simulink model "QArm_Workspace_MB_2"  (R2021a)
settings: Solver=ode4  StartTime=0.0  StopTime=inf  FixedStep=1/1000  RelTol=1e-3  EnableMultiTasking=on
model workspace (MAT data in the model file):
  cameraStepSize : Simulink.Parameter (value not decoded)
  mainStepSize : Simulink.Parameter (value not decoded)
symbols that are objects in the model workspace (value not decoded): cameraStepSize, mainStepSize
undefined symbols (not defined in the file): interleaved, RGB
libraries: quarc_library x12, simulink x3
(part 2 of 3)

== system QArm_Workspace_MB_2/Virtual QArm/Manipulator Joint Plants/Base Joint 1 ==
  note: v = IR + kv omega
      | Tau = i kt
      | Tau = J theta_dot_dot + b * omega + k *sign(omega)
  Voltage : Inport
  tau_g (Nm) : Inport  Port=2
  reset : Inport  Port=3
  Constant : Constant  Value=0.001*272.5
  Divide : Product  Inputs=*/
  Divide{1,3..5} (4 alike) : Product  Inputs=**
  Divide2 : Product  Inputs=*/
  Integrator1 : Integrator  ExternalReset=rising  LimitOutput=on  UpperSaturationLimit=pi*[170]/180  LowerSaturationLimit=pi*[-170]/180
  Integrator2 : Integrator  LimitOutput=on  UpperSaturationLimit=pi/2  LowerSaturationLimit=-pi/2
  J * GR^2 : Constant  Value=272.5^2*0.65e-05
  R : Constant
  Sign : Signum
  Subtract{,1..3} (4 alike) : Sum  Inputs=+-
  b * GR : Constant  Value=0.0005*272.5
  kt * GR : Constant  Value=0.01495*272.5
  kv * GR : Constant  Value=0.0135*272.5
  phi (rad) : Outport  VectorParamsAs1DForOutWhenUnconnected=off
  phi_dot (rad/s) : Outport  Port=2  VectorParamsAs1DForOutWhenUnconnected=off
  current (A) : Outport  Port=3  VectorParamsAs1DForOutWhenUnconnected=off
  wires:
  R/1 -> Divide/2
  Subtract/1 -> Divide/1
  kt * GR/1 -> Divide1/2
  Divide/1 -> current (A)/1, Divide1/1
  Divide3/1 -> Subtract/2
  Divide1/1 -> Subtract1/1
  J * GR^2/1 -> Divide2/2
  Voltage/1 -> Subtract/1
  kv * GR/1 -> Divide3/2
  b * GR/1 -> Divide4/2
  Integrator1/1 -> phi (rad)/1  "phi"
  Divide2/1 -> Integrator2/1
  Divide4/1 -> Subtract1/2
  Constant/1 -> Divide5/2
  Sign/1 -> Divide5/1
  Integrator2/1 -> Sign/1, Divide4/1, Divide3/1, Integrator1/1, phi_dot (rad/s)/1  "Speed"
  Subtract1/1 -> Subtract2/1
  Divide5/1 -> Subtract2/2
  Subtract2/1 -> Subtract3/1
  Subtract3/1 -> Divide2/1
  tau_g (Nm)/1 -> Subtract3/2
  reset/1 -> Integrator1/2

== system QArm_Workspace_MB_2/Virtual QArm/Manipulator Joint Plants/Elbow Joint 3 ==
  Voltage : Inport
  tau_g (Nm) : Inport  Port=2
  reset : Inport  Port=3
  Constant : Constant  Value=0.001*272.5
  Divide : Product  Inputs=*/
  Divide{1,3..5} (4 alike) : Product  Inputs=**
  Divide2 : Product  Inputs=*/
  Integrator1 : Integrator  ExternalReset=rising  LimitOutput=on  UpperSaturationLimit=pi*[75]/180  LowerSaturationLimit=pi*[-95]/180
  Integrator2 : Integrator  LimitOutput=on  UpperSaturationLimit=pi/2  LowerSaturationLimit=-pi/2
  J * GR^2 : Constant  Value=272.5^2*0.75e-05
  R : Constant  Value=5
  Sign : Signum
  Subtract{,1..3} (4 alike) : Sum  Inputs=+-
  b * GR : Constant  Value=0.02*272.5
  kt * GR : Constant  Value=0.1*272.5
  kv * GR : Constant  Value=0.01*272.5
  phi (rad) : Outport  VectorParamsAs1DForOutWhenUnconnected=off
  phi_dot (rad/s) : Outport  Port=2  VectorParamsAs1DForOutWhenUnconnected=off
  current (A) : Outport  Port=3  VectorParamsAs1DForOutWhenUnconnected=off
  wires:
  R/1 -> Divide/2
  Subtract/1 -> Divide/1
  kt * GR/1 -> Divide1/2
  Divide/1 -> current (A)/1, Divide1/1
  Integrator2/1 -> Divide4/1, Divide3/1, Sign/1, phi_dot (rad/s)/1, Integrator1/1  "Speed"
  Divide3/1 -> Subtract/2
  Divide1/1 -> Subtract1/1
  J * GR^2/1 -> Divide2/2
  Subtract1/1 -> Subtract2/1
  Voltage/1 -> Subtract/1
  kv * GR/1 -> Divide3/2
  b * GR/1 -> Divide4/2
  Integrator1/1 -> phi (rad)/1  "phi"
  Divide2/1 -> Integrator2/1
  Divide4/1 -> Subtract1/2
  Divide5/1 -> Subtract2/2
  Constant/1 -> Divide5/2
  Sign/1 -> Divide5/1
  Subtract3/1 -> Divide2/1
  Subtract2/1 -> Subtract3/1
  tau_g (Nm)/1 -> Subtract3/2
  reset/1 -> Integrator1/2

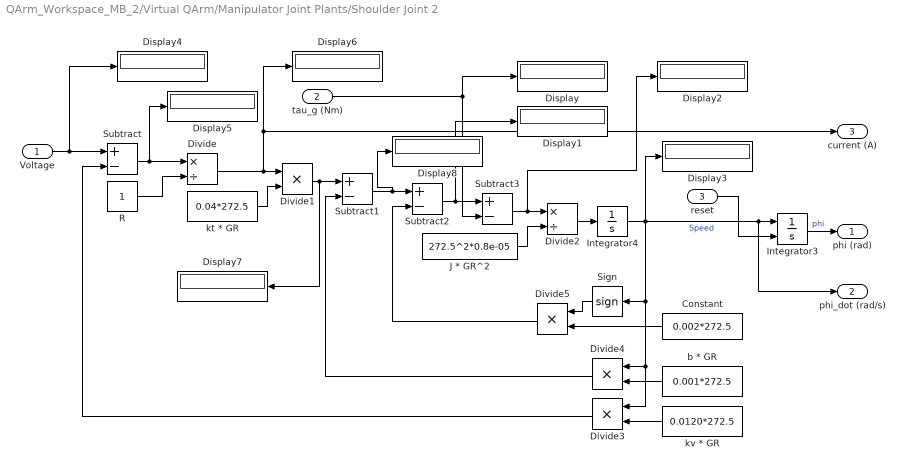
== system QArm_Workspace_MB_2/Virtual QArm/Manipulator Joint Plants/Shoulder Joint 2 ==
  Voltage : Inport
  tau_g (Nm) : Inport  Port=2
  reset : Inport  Port=3
  Constant : Constant  Value=0.002*272.5
  Display{,1..8} (9 alike) : Display
  Divide : Product  Inputs=*/
  Divide{1,3..5} (4 alike) : Product  Inputs=**
  Divide2 : Product  Inputs=*/
  Integrator3 : Integrator  ExternalReset=rising  LimitOutput=on  UpperSaturationLimit=pi*[85]/180  LowerSaturationLimit=pi*[-85]/180
  Integrator4 : Integrator  LimitOutput=on  UpperSaturationLimit=pi/2  LowerSaturationLimit=-pi/2
  J * GR^2 : Constant  Value=272.5^2*0.8e-05
  R : Constant
  Sign : Signum
  Subtract{,1..3} (4 alike) : Sum  Inputs=+-
  b * GR : Constant  Value=0.001*272.5
  kt * GR : Constant  Value=0.04*272.5
  kv * GR : Constant  Value=0.0120*272.5
  phi (rad) : Outport  VectorParamsAs1DForOutWhenUnconnected=off
  phi_dot (rad/s) : Outport  Port=2  VectorParamsAs1DForOutWhenUnconnected=off
  current (A) : Outport  Port=3  VectorParamsAs1DForOutWhenUnconnected=off
  wires:
  Divide4/1 -> Subtract1/2
  Divide2/1 -> Integrator4/1
  Integrator3/1 -> phi (rad)/1  "phi"
  b * GR/1 -> Divide4/2
  kv * GR/1 -> Divide3/2
  Voltage/1 -> Display4/1, Subtract/1
  Subtract1/1 -> Display8/1, Subtract2/1
  J * GR^2/1 -> Divide2/2
  Divide1/1 -> Subtract1/1, Display7/1
  Divide3/1 -> Subtract/2
  Divide/1 -> Divide1/1, Display6/1, current (A)/1
  kt * GR/1 -> Divide1/2
  Subtract/1 -> Display5/1, Divide/1
  R/1 -> Divide/2
  Constant/1 -> Divide5/2
  Sign/1 -> Divide5/1
  Integrator4/1 -> Display3/1, Integrator3/1, phi_dot (rad/s)/1, Sign/1, Divide3/1, Divide4/1  "Speed"
  Divide5/1 -> Subtract2/2
  Subtract3/1 -> Display2/1, Divide2/1
  Subtract2/1 -> Display1/1, Subtract3/1
  tau_g (Nm)/1 -> Subtract3/2, Display/1
  reset/1 -> Integrator3/2

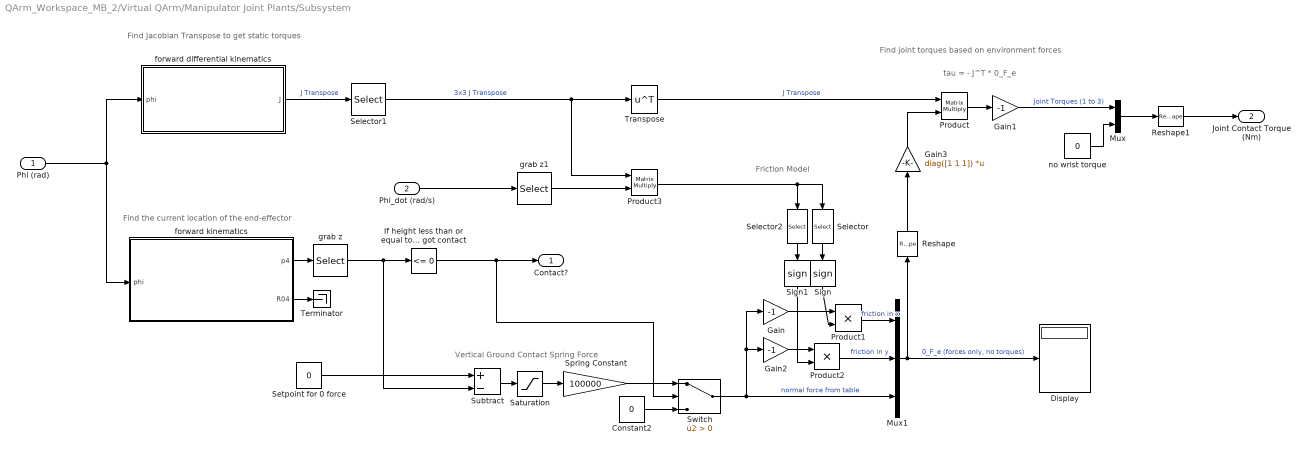
== system QArm_Workspace_MB_2/Virtual QArm/Manipulator Joint Plants/Subsystem ==
  note: Friction Model
  note: Vertical Ground Contact Spring Force
  note: Find joint torques based on environment forces
  note: Find Jacobian Transpose to get static torques
  note: Find the current location of the end-effector
  note: tau = - J^T * 0_F_e
  Phi (rad) : Inport  PortDimensions=4
  Phi_dot (rad/s) : Inport  Port=2  PortDimensions=4
  Constant2 : Constant  Value=0
  Display : Display
  Gain : Gain  Gain=-1
  Gain1 : Gain  Gain=-1
  Gain2 : Gain  Gain=-1
  Gain3 : Gain  Gain=diag([1 1 1])  Multiplication=Matrix(K*u)
  "If height less than or equal to 0, then we've got contact" : simulink/Logic and Bit Operations/Compare To Constant  relop=<=  const=0  OutDataTypeStr=boolean
  Mux : Mux  Inputs=2
  Mux1 : Mux  Inputs=3
  Product : Product  Multiplication=Matrix(*)
  Product1 : Product
  Product2 : Product
  Product3 : Product  Multiplication=Matrix(*)
  Reshape : Reshape  OutputDimensionality=Column vector (2-D)
  Reshape1 : Reshape
  Saturation : Saturate  UpperLimit=Inf  LowerLimit=0
  Selector : Selector  InputPortWidth=3  IndexOptions=Index vector (dialog)  Indices=1  OutputSizes=1
  Selector1 : Selector  NumberOfDimensions=2  InputPortWidth=3  IndexOptions=Index vector (dialog),Index vector (dialog)  Indices=[1:3],[1:3]  OutputSizes=1,1
  Selector2 : Selector  InputPortWidth=3  IndexOptions=Index vector (dialog)  Indices=2  OutputSizes=1
  Setpoint for 0 force : Constant  Value=0
  Sign : Signum
  Sign1 : Signum
  Spring Constant : Gain  Gain=100000
  Subtract : Sum  Inputs=+-
  Switch : Switch  Criteria=u2 > Threshold
  Terminator : Terminator
  Transpose : Math  Operator=transpose  SignedPower=on  SaturateOnIntegerOverflow=on
  forward differential kinematics : MATLAB Function  TreatAsAtomicUnit=on
  forward kinematics : MATLAB Function  TreatAsAtomicUnit=on
  grab z : Selector  InputPortWidth=3  IndexOptions=Index vector (dialog)  Indices=3  OutputSizes=1
  grab z1 : Selector  InputPortWidth=4  IndexOptions=Index vector (dialog)  Indices=[1:3]  OutputSizes=1
  no wrist torque : Constant  Value=0
  Contact? : Outport  VectorParamsAs1DForOutWhenUnconnected=off
  Joint Contact Torque (Nm) : Outport  Port=2  VectorParamsAs1DForOutWhenUnconnected=off
  wires:
  forward kinematics/1(p4) -> grab z/1
  forward kinematics/2(R04) -> Terminator/1
  grab z/1 -> "If height less than or equal to 0, then we've got contact"/1, Subtract/2
  forward differential kinematics/1(J) -> Selector1/1  "J Transpose"
  Mux1/1 -> Reshape/1, Display/1  "0_F_e (forces only, no torques)"
  Selector1/1 -> Product3/1, Transpose/1  "3x3 J Transpose"
  Product/1 -> Gain1/1
  no wrist torque/1 -> Mux/2
  Mux/1 -> Reshape1/1
  Gain1/1 -> Mux/1  "Joint Torques (1 to 3)"
  Switch/1 -> Mux1/3, Gain2/1, Gain/1  "normal force from table"
  Product2/1 -> Mux1/2  "friction in y"
  "If height less than or equal to 0, then we've got contact"/1 -> Contact?/1, Switch/2
  Constant2/1 -> Switch/3
  Spring Constant/1 -> Switch/1
  Setpoint for 0 force/1 -> Subtract/1
  Subtract/1 -> Saturation/1
  Phi (rad)/1 -> forward differential kinematics/1(phi), forward kinematics/1(phi)
  Reshape/1 -> Gain3/1
  Reshape1/1 -> Joint Contact Torque (Nm)/1
  Product1/1 -> Mux1/1  "friction in x"
  Saturation/1 -> Spring Constant/1
  Phi_dot (rad/s)/1 -> grab z1/1
  Product3/1 -> Selector2/1, Selector/1
  Gain/1 -> Product1/1
  Gain2/1 -> Product2/1
  Selector/1 -> Sign/1
  Selector2/1 -> Sign1/1
  Gain3/1 -> Product/2
  Sign/1 -> Product1/2
  Sign1/1 -> Product2/2
  Transpose/1 -> Product/1  "J Transpose"
  grab z1/1 -> Product3/2

== system QArm_Workspace_MB_2/Virtual QArm/Manipulator Joint Plants/Wrist Joint 4 ==
  Voltage : Inport
  tau_g (Nm) : Inport  Port=2
  reset : Inport  Port=3
  Constant : Constant  Value=0.001*272.5
  Divide : Product  Inputs=*/
  Divide{1,3..5} (4 alike) : Product  Inputs=**
  Divide2 : Product  Inputs=*/
  Integrator3 : Integrator  ExternalReset=rising  LimitOutput=on  UpperSaturationLimit=pi*[167.5]/180  LowerSaturationLimit=pi*[-167.5]/180
  Integrator4 : Integrator  LimitOutput=on  UpperSaturationLimit=pi  LowerSaturationLimit=-pi
  J * GR^2 : Constant  Value=272.5^2*0.5e-05
  R : Constant  Value=6
  Sign : Signum
  Subtract{,1..3} (4 alike) : Sum  Inputs=+-
  b * GR : Constant  Value=0.001*272.5
  kt * GR : Constant  Value=0.3*272.5
  kv * GR : Constant  Value=0.0095*272.5
  phi (rad) : Outport  VectorParamsAs1DForOutWhenUnconnected=off
  phi_dot (rad/s) : Outport  Port=2  VectorParamsAs1DForOutWhenUnconnected=off
  current (A) : Outport  Port=3  VectorParamsAs1DForOutWhenUnconnected=off
  wires:
  Divide4/1 -> Subtract1/2
  Divide2/1 -> Integrator4/1
  Integrator3/1 -> phi (rad)/1  "phi"
  b * GR/1 -> Divide4/2
  kv * GR/1 -> Divide3/2
  Voltage/1 -> Subtract/1
  Subtract1/1 -> Subtract2/1
  J * GR^2/1 -> Divide2/2
  Divide1/1 -> Subtract1/1
  Divide3/1 -> Subtract/2
  Divide/1 -> Divide1/1, current (A)/1
  kt * GR/1 -> Divide1/2
  Subtract/1 -> Divide/1
  R/1 -> Divide/2
  Sign/1 -> Divide5/1
  Constant/1 -> Divide5/2
  Integrator4/1 -> Integrator3/1, phi_dot (rad/s)/1, Sign/1, Divide3/1, Divide4/1  "Speed"
  Divide5/1 -> Subtract2/2
  Subtract3/1 -> Divide2/1
  Subtract2/1 -> Subtract3/1
  tau_g (Nm)/1 -> Subtract3/2
  reset/1 -> Integrator3/2

== matlab function QArm_Workspace_MB_2/To//From Simulation/MATLAB Function4 ==
  settings: updateMethod=DISCRETE  sampleTime=mainStepSize
  data: Packet output size=65537; ServerState input; SendStateUpdate input; Enable output; DeviceNumber input; Clock input; Threshold input
function [Packet,Enable] = QArmApplicationWorkspaceMakeVideoPacketData(ServerState, SendStateUpdate, DeviceNumber, Clock, Threshold) 

% Be sure to set the maximum signal size of the variable size Packet port 
% in Simulink->Edit Data of the editor window.  Size should be 65537 or
% larger to ensure that the stream server generates a 4 byte packet size.

%% Setup
persistent LastServerState;
persistent timeLastSend;
persistent readyToSend;

if isempty(LastServerState)
    LastServerState = uint8(0);
    readyToSend = uint8(0);
    timeLastSend = -Threshold;
end

Enable = 0;
Packet = uint8([]);

%% On connection
if ((ServerState == 2) && (LastServerState ~= 2))
    Packet = QArmMakeRGBRawRequestContainer(DeviceNumber);
    Packet = [Packet; QArmMakeDepthRawRequestContainer(DeviceNumber)];
end

%% Send new State Container
% Previous state processed, send a new one
if (SendStateUpdate)
    readyToSend = uint8(1);
end

if readyToSend && ((Clock - timeLastSend) > Threshold)
    Packet = QArmMakeRGBRawRequestContainer(DeviceNumber);
    Packet = [Packet; QArmMakeDepthRawRequestContainer(DeviceNumber)];   
    readyToSend = uint8(0);
    timeLastSend = Clock;
end


%% Transmit
% If we have data to send, enable the transmit
PacketLength = length(Packet);

if (PacketLength > 0)
    % Add magic byte.  This is just for error handling and isn't typically
    % required in simulink, but useful in lower-level languages like Python
    Packet = [uint8(123); Packet];
    
    Enable = 1; 
end

LastServerState = ServerState;

== matlab function QArm_Workspace_MB_2/Virtual QArm/Manipulator Joint Plants/Gravitational Torque ==
  data: phi input; G output; payload input
function G  = fcn(phi, payload)

%% Manipulator Parameters and Initialization

% Manipulator natural link lengths
L1 = 0.1400;
L2 = 0.3500;
L3 = 0.0500;
L4 = 0.2500;
L5 = 0.1500;

% Manipulator bend angle at joint 3
beta = atan(L3/L2);

% Manipulator mathematical link lenghts
l1 = L1;
l2 = sqrt(L2^2 + L3^2);
l3 = L4 + L5;

% Phi-space to Theta-space
theta = phi;
theta(1) = phi(1);
theta(2) = phi(2) + beta - pi/2;
theta(3) = phi(3) - beta;
theta(4) = phi(4);

%% Dynamic Parameters (Inertias and Masses)

% Masses
mT = 1.75;
m1 = 0.3*mT*l1 / (l1 + l2 + l3);
m2 = mT*l2 / (l1 + l2 + l3);
m3 = mT*L4 / (l1 + l2 + l3);
m4 = mT*L5 / (l1 + l2 + l3);
mL = payload;

% Center of mass locations
% Note: lc1 is unused as the first link does not move linearly (v_1 = 0)
lc2 = l2/2;
lc3 = L4/2;
lc4 = L5/2;

%% Gravity Matrix

g = 9.81;
G2 = -g*(m2*(l2 - lc2)*cos(theta(2)) + m3*(l2*cos(theta(2)) - lc3*sin(theta(2)+theta(3))) + m4*(l2*cos(theta(2)) - (l3 - lc4)*sin(theta(2)+theta(3))) + mL*(l2*cos(theta(2)) - l3*sin(theta(2)+theta(3))) );
G3 = g*(m3*lc3*sin(theta(2)+theta(3)) + m4*(l3 - lc4)*sin(theta(2)+theta(3)) + mL*l3*sin(theta(2)+theta(3)) );

G = [0; G2; G3; 0];

== matlab function QArm_Workspace_MB_2/To//From Simulation/MATLAB Function5 ==
  data: Receive input; RequestServerUpdate output; NewRGB output; New input; RGB output; NewDepth output; Depth output
function [RequestServerUpdate, NewRGB, RGB, NewDepth, Depth]  = QArmApplicationWorkspaceDecodeVideoPacket(Receive, New)

%% Setup

num_columns = 1280;
num_rows = 720;

RGB = zeros(num_rows*num_columns*3, 1, 'uint8');
Depth = zeros(num_rows*num_columns*3, 1, 'uint8');

NewRGB = 0;
NewDepth = 0;

RequestServerUpdate = 0;
PacketSize = length(Receive);

%Packet > 0, new data, and magic number in first index
if ((PacketSize > 0) && (New == 1) && (Receive(1) == uint8(123)))
    
    %skip magic number
    Index = int32(2);
    
    while(Index <= PacketSize)
       
        %% Get container details
        ContainerSize = typecast(uint8(flip(Receive(Index:Index+3))), 'int32');
        DeviceID = typecast(uint8(flip(Receive(Index+4:Index+7))), 'int32');
        DeviceNum = typecast(uint8(flip(Receive(Index+8:Index+12))), 'int32');
        DeviceFunction = uint8(Receive(Index+12));
        PayloadStart = Index+13;
        PayloadEnd = Index+ContainerSize-1;
        
        %% Pass container to appropriate decoding function
        if (DeviceID == 10) %is this a QArm container?
            
            if (DeviceFunction == 103) % Pull out RGB payload for external processing
                RGBSize = typecast(uint8(flip(Receive(PayloadStart:PayloadStart+3))), 'int32');
                RGB(1:num_rows*num_columns*3) = Receive(PayloadStart+4:PayloadStart+4+num_rows*num_columns*3);
                NewRGB = 1;
                RequestServerUpdate = 1;
                
            elseif (DeviceFunction == 113) % Pull out Depth payload for external processing
                DepthSize = typecast(uint8(flip(Receive(PayloadStart:PayloadStart+3))), 'int32');
                Depth(1:num_rows*num_columns*3) = Receive(PayloadStart+4:PayloadStart+4+num_rows*num_columns*3);
                NewDepth = 1;
                RequestServerUpdate = 1;
            end
        end
        
        
        
        %% Process next container if any data is left.
        Index = Index+ContainerSize;
    end


end

== matlab function QArm_Workspace_MB_2/To//From Simulation/MATLAB Function3 ==
  data: Receive input size=65537; RequestServerUpdate output; NewRGB output; New input; RGB output size=65537; NewDepth output; Depth output size=65537
function [RequestServerUpdate, NewRGB, RGB, NewDepth, Depth]  = QArmApplicationWorkspaceDecodeVideoPacket(Receive, New)

%% Setup
RGB = uint8([]);
Depth = uint8([]);

NewRGB = 0;
NewDepth = 0;

RequestServerUpdate = 0;
PacketSize = length(Receive);

% Packet > 0, new data, and magic number in first index
if ((PacketSize > 0) && (New == 1) && (Receive(1) == uint8(123)))
    
    %skip magic number
    Index = int32(2);
    
    while(Index <= PacketSize)
       
                %% Get container details
        ContainerSize = typecast(uint8(flip(Receive(Index:Index+3))), 'int32');
        DeviceID = typecast(uint8(flip(Receive(Index+4:Index+7))), 'int32');
        DeviceNum = typecast(uint8(flip(Receive(Index+8:Index+11))), 'int32');
        DeviceFunction = uint8(Receive(Index+12));
        PayloadStart = Index+13;
        PayloadEnd = Index+ContainerSize-1;
        
        %% Pass container to appropriate decoding function
        if (DeviceID == 10) %is this a QArm container?
            
            if (DeviceFunction == 2) % Pull out RGB payload for external processing
                RequestServerUpdate = 1;
            
            elseif (DeviceFunction == 101) % Pull out RGB payload for external processing
                RGBSize = typecast(uint8(flip(Receive(PayloadStart:PayloadStart+3))), 'int32');
                RGB = Receive(PayloadStart+4:PayloadEnd);
                NewRGB = 1;
                RequestServerUpdate = 1;
                
            elseif (DeviceFunction == 111) % Pull out Depth payload for external processing
                DepthSize = typecast(uint8(flip(Receive(PayloadStart:PayloadStart+3))), 'int32');
                Depth = Receive(PayloadStart+4:PayloadEnd);
                NewDepth = 1;
                RequestServerUpdate = 1;
            end
        end
        
        
        
        %% Process next container if any data is left.
        Index = Index+ContainerSize;
    end


end

== matlab function QArm_Workspace_MB_2/To//From Simulation/Collision/inverse kinematics ==
  data: p input; gamma input; phi_optimal output; phi_prev input
function phi_optimal  = qarmInverseKinematics(p, gamma, phi_prev)

%% QUANSER_ARM_IPK
% v 4.0 - 4th June 2020

% REFERENCE: 
% Chapter 4. Inverse Kinematics
% Robot Dynamics and Control 
% Spong, Vidyasagar
% 1989

% INPUTS:
% p        : end-effector position vector expressed in base frame {0}
% gamma    : wrist rotation angle gamma

% OUTPUTS:
% phi_optimal : Best solution depending on phi_prev
% phi         : All four Inverse Kinematics solutions as a 4x4 matrix. 
%               Each col is a solution.

%% Manipulator parameters:
L1 = 0.1400;
L2 = 0.3500;
L3 = 0.0500;
L4 = 0.2500;
L5 = 0.1500;
beta = atan(L3/L2);

%% Alternate parameters
lambda1 = L1;
lambda2 = sqrt(L2^2 + L3^2);
lambda3 = L4 + L5;

%% Initialization
theta   = zeros(4, 4);
phi = zeros(4, 4);

%% Joint angle 2 and 3: 
% Equations:
    % lambda2 cos(theta2) + (-lambda3) sin(theta2 + theta3) = sqrt(x^2 + y^2)
    %   A     cos( 2    ) +     C      sin(   2   +    3  ) =    D
    
    % lambda2 sin(theta2) - (-lambda3) cos(theta2 + theta3) = lambda1 - z
    %   A     sin( 2    ) -     C      cos(   2   +    3  ) =    H

% Solution:
    A = lambda2;
    C = -lambda3;
    H =  lambda1 - p(3);
    D1 = -sqrt(p(1)^2 + p(2)^2);
    D2 = sqrt(p(1)^2 + p(2)^2);
    F = (D1^2 + H^2 - A^2 - C^2)/(2*A);

    theta(3,1) = 2*atan2( C + sqrt(C^2 - F^2) , F );
	theta(3,2) = 2*atan2( C - sqrt(C^2 - F^2) , F );
    theta(3,3) = 2*atan2( C + sqrt(C^2 - F^2) , F );
	theta(3,4) = 2*atan2( C - sqrt(C^2 - F^2) , F );

    M = A + C*sin(theta(3,1));
    N = -C*cos(theta(3,1));
    cos_term = (D1*M + H*N)/(M^2 + N^2);
    sin_term = (H - N*cos_term)/(M);
    theta(2,1) = atan2(sin_term, cos_term);

    M = A + C*sin(theta(3,2));
    N = -C*cos(theta(3,2));
    cos_term = (D1*M + H*N)/(M^2 + N^2);
    sin_term = (H - N*cos_term)/(M);
    theta(2,2) = atan2(sin_term, cos_term);

    M = A + C*sin(theta(3,3));
    N = -C*cos(theta(3,3));
    cos_term = (D2*M + H*N)/(M^2 + N^2);
    sin_term = (H - N*cos_term)/(M);
    theta(2,3) = atan2(sin_term, cos_term);

    M = A + C*sin(theta(3,4));
    N = -C*cos(theta(3,4));
    cos_term = (D2*M + H*N)/(M^2 + N^2);
    sin_term = (H - N*cos_term)/(M);
    theta(2,4) = atan2(sin_term, cos_term);


%% Joint angle 1:
% Equation:
    % y / x = tan(theta1);

% Solution
    theta(1,1) = atan2( p(2)/( lambda2 * cos( theta(2,1) ) - lambda3 * sin( theta(2,1) + theta(3,1) ) ) , p(1)/(  lambda2 * cos( theta(2,1) ) - lambda3 * sin( theta(2,1) + theta(3,1) )  ) );
    theta(1,2) = atan2( p(2)/( lambda2 * cos( theta(2,2) ) - lambda3 * sin( theta(2,2) + theta(3,2) ) ) , p(1)/(  lambda2 * cos( theta(2,2) ) - lambda3 * sin( theta(2,2) + theta(3,2) )  ) );
    theta(1,3) = atan2( p(2)/( lambda2 * cos( theta(2,3) ) - lambda3 * sin( theta(2,3) + theta(3,3) ) ) , p(1)/(  lambda2 * cos( theta(2,3) ) - lambda3 * sin( theta(2,3) + theta(3,3) )  ) );
    theta(1,4) = atan2( p(2)/( lambda2 * cos( theta(2,4) ) - lambda3 * sin( theta(2,4) + theta(3,4) ) ) , p(1)/(  lambda2 * cos( theta(2,4) ) - lambda3 * sin( theta(2,4) + theta(3,4) )  ) );
    
%% Remap theta back to phi
% phi(1) = theta(1);
% phi(2) = theta(2) - beta + pi/2;
% phi(3) = theta(3) + beta;
% phi(4) = theta(4);

phi(1,:) = theta(1,:);
phi(2,:) = theta(2,:) - beta + pi/2;
phi(3,:) = theta(3,:) + beta;
phi(4,:) = gamma;

phi = mod(phi + pi, 2*pi) - pi;

phi_optimal = phi(:,1);
if norm(phi_optimal - phi_prev) > norm(phi(:,2) - phi_prev)
    phi_optimal = phi(:,2);
end
if norm(phi_optimal - phi_prev) > norm(phi(:,3) - phi_prev)
    phi_optimal = phi(:,3);
end
if norm(phi_optimal - phi_prev) > norm(phi(:,4) - phi_prev)
    phi_optimal = phi(:,4);
end

end

== matlab function QArm_Workspace_MB_2/To//From Simulation/Collision/MATLAB Function ==
  settings: updateMethod=DISCRETE
  data: user_phi input; user_p input; position_cmd output; target input; actual input; R04 input; where output; offset input
function [position_cmd, where] = fcn(user_phi, user_p, target, actual, R04, offset)

persistent state
persistent phi
persistent p
persistent actual_hold
change = 0; collision = 0;

if isempty(state)
    state = 1;
    phi = user_phi;
    actual_hold = actual;
end

if norm(user_phi-phi, 2) > 0.001
    change = 1;
end

if norm(target-actual, 2) > 0.001
    collision = 1;
end

switch state
    case 1
        if collision
            state = 2;
        else
            state = 1;
        end
        p = user_p;
        
    case 2
        state = 3;
        actual_hold = actual;
        p = actual_hold - R04*offset;
        
    case 3
        if change
            state = 1;
        else
            state = 3;
        end      
        
        p = actual_hold - R04*offset;
        
    otherwise
        p = user_p;
end

phi = user_phi;
position_cmd = p;
where = state;

== matlab function QArm_Workspace_MB_2/To//From Simulation/Collision/forward kinematics1 ==
  data: phi input; p4 output; R04 output
function [p4, R04] = qarmForwardKinematics(phi)

%% QUANSER_ARM_FPK
% v 4.0 - 4th June 2020

% REFERENCE: 
% Chapter 3. Forward Kinematics
% Robot Dynamics and Control 
% Spong, Vidyasagar
% 1989

% INPUTS:
% phi     : Alternate joint angles vector 4 x 1

% OUTPUTS:
% p4      : End-effector frame {4} position vector expressed in base frame {0}
% R04     : rotation matrix from end-effector frame {4} to base frame {0}

%% Manipulator parameters:
L1 = 0.1400;
L2 = 0.3500;
L3 = 0.0500;
L4 = 0.2500;
L5 = 0.1500;

%% Alternate parameters
l1 = L1;
l2 = sqrt(L2^2 + L3^2);
l3 = L4 + L5;
beta = atan(L3/L2);

%% From phi space to theta space 
theta = phi;
theta(1) = phi(1);
theta(2) = phi(2) + beta - pi/2;
theta(3) = phi(3) - beta;
theta(4) = phi(4);

%% Transformation matrices for all frames:

% T{i-1}{i} = quanser_arm_DH(  a, alpha,  d,     theta );
        T01 = quanser_arm_DH(  0, -pi/2, l1,  theta(1) );
        T12 = quanser_arm_DH( l2,     0,  0,  theta(2) );
        T23 = quanser_arm_DH(  0, -pi/2,  0,  theta(3) );
        T34 = quanser_arm_DH(  0,     0, l3,  theta(4) );

        T02 = T01*T12;
        T03 = T02*T23;
        T04 = T03*T34;

%% Position of end-effector Transformation

% Extract the Position vector 
% p1   = T01(1:3,4);
% p2   = T02(1:3,4);
% p3   = T03(1:3,4);
p4   = T04(1:3,4);

% Extract the Rotation matrix
% R01 = T01(1:3,1:3);
% R02 = T02(1:3,1:3);
% R03 = T03(1:3,1:3);
R04 = T04(1:3,1:3);

end

function T = quanser_arm_DH(a,alpha,d,theta)

%% QUANSER_ARM_DH
% v 1.0 - 26th March 2019

% REFERENCE: 
% Chapter 3. Forward and Inverse Kinematics
% Robot Modeling and Control 
% Spong, Hutchinson, Vidyasagar
% 2006

% INPUTS:
% a       :   translation  : along : x_{i}   : from : z_{i-1} : to : z_{i}
% alpha   :      rotation  : about : x_{i}   : from : z_{i-1} : to : z_{i}
% d       :   translation  : along : z_{i-1} : from : x_{i-1} : to : x_{i}
% theta   :      rotation  : about : z_{i-1} : from : x_{i-1} : to : x_{i}
% NOTE: Standard DH Parameters

% OUTPUTS:
% T       : transformation                   : from :     {i} : to : {i-1}

%%
% Rotation Transformation about z axis by theta
T_R_z = [cos(theta) -sin(theta) 0 0;
         sin(theta)  cos(theta) 0 0;
                  0           0 1 0;
                  0           0 0 1];
     
% Translation Transformation along z axis by d
T_T_z = [1 0 0 0;
         0 1 0 0;
         0 0 1 d;
         0 0 0 1];

% Translation Transformation along x axis by a
T_T_x = [1 0 0 a;
         0 1 0 0;
         0 0 1 0;
         0 0 0 1];

% Rotation Transformation about x axis by alpha
T_R_x = [1          0           0 0;
         0 cos(alpha) -sin(alpha) 0;
         0 sin(alpha)  cos(alpha) 0;
         0          0           0 1];

% For a transformation FROM frame {i} TO frame {i-1}: A
T = T_R_z*T_T_z*T_T_x*T_R_x;

end

== matlab function QArm_Workspace_MB_2/To//From Simulation/Collision (Archive)/MATLAB Function ==
  data: user_phi input; user_p input; position_cmd output; target input; actual input; R04 input
function position_cmd = fcn(user_phi, user_p, target, actual, R04)

persistent state
persistent phi
persistent p
persistent actual_hold
change = 0; collision = 0;

if isempty(state)
    state = 1;
    phi = user_phi;
    p = user_p;
    actual_hold = actual;
end

if user_phi ~= phi
    change = 1;
end

if target ~= actual
    collision = 1;
end

switch state
    case 1
        if collision
            state = 2;
        else
            state = 1;
        end
        p = user_p;
        
    case 2
        state = 3;
        actual_hold = actual;
        p = actual_hold - R04*[-0.0256;0;-0.1162];
        
    case 3
        if change
            state = 1;
        else
            state = 3;
        end      
        
        p = actual_hold - R04*[-0.0256;0;-0.1162];
        
    otherwise
        p = user_p;
end

phi = user_phi;
position_cmd = p;

== matlab function QArm_Workspace_MB_2/To//From Simulation/Collision (Archive)/forward kinematics ==
  data: phi input; p4 output; R04 output
function [p4, R04] = qarmForwardKinematics(phi)

%% QUANSER_ARM_FPK
% v 4.0 - 4th June 2020

% REFERENCE: 
% Chapter 3. Forward Kinematics
% Robot Dynamics and Control 
% Spong, Vidyasagar
% 1989

% INPUTS:
% phi     : Alternate joint angles vector 4 x 1

% OUTPUTS:
% p4      : End-effector frame {4} position vector expressed in base frame {0}
% R04     : rotation matrix from end-effector frame {4} to base frame {0}

%% Manipulator parameters:
L1 = 0.1400;
L2 = 0.3500;
L3 = 0.0500;
L4 = 0.2500;
L5 = 0.1500;

%% Alternate parameters
l1 = L1;
l2 = sqrt(L2^2 + L3^2);
l3 = L4 + L5;
beta = atan(L3/L2);

%% From phi space to theta space 
theta = phi;
theta(1) = phi(1);
theta(2) = phi(2) + beta - pi/2;
theta(3) = phi(3) - beta;
theta(4) = phi(4);

%% Transformation matrices for all frames:

% T{i-1}{i} = quanser_arm_DH(  a, alpha,  d,     theta );
        T01 = quanser_arm_DH(  0, -pi/2, l1,  theta(1) );
        T12 = quanser_arm_DH( l2,     0,  0,  theta(2) );
        T23 = quanser_arm_DH(  0, -pi/2,  0,  theta(3) );
        T34 = quanser_arm_DH(  0,     0, l3,  theta(4) );

        T02 = T01*T12;
        T03 = T02*T23;
        T04 = T03*T34;

%% Position of end-effector Transformation

% Extract the Position vector 
% p1   = T01(1:3,4);
% p2   = T02(1:3,4);
% p3   = T03(1:3,4);
p4   = T04(1:3,4);

% Extract the Rotation matrix
% R01 = T01(1:3,1:3);
% R02 = T02(1:3,1:3);
% R03 = T03(1:3,1:3);
R04 = T04(1:3,1:3);

end

function T = quanser_arm_DH(a,alpha,d,theta)

%% QUANSER_ARM_DH
% v 1.0 - 26th March 2019

% REFERENCE: 
% Chapter 3. Forward and Inverse Kinematics
% Robot Modeling and Control 
% Spong, Hutchinson, Vidyasagar
% 2006

% INPUTS:
% a       :   translation  : along : x_{i}   : from : z_{i-1} : to : z_{i}
% alpha   :      rotation  : about : x_{i}   : from : z_{i-1} : to : z_{i}
% d       :   translation  : along : z_{i-1} : from : x_{i-1} : to : x_{i}
% theta   :      rotation  : about : z_{i-1} : from : x_{i-1} : to : x_{i}
% NOTE: Standard DH Parameters

% OUTPUTS:
% T       : transformation                   : from :     {i} : to : {i-1}

%%
% Rotation Transformation about z axis by theta
T_R_z = [cos(theta) -sin(theta) 0 0;
         sin(theta)  cos(theta) 0 0;
                  0           0 1 0;
                  0           0 0 1];
     
% Translation Transformation along z axis by d
T_T_z = [1 0 0 0;
         0 1 0 0;
         0 0 1 d;
         0 0 0 1];

% Translation Transformation along x axis by a
T_T_x = [1 0 0 a;
         0 1 0 0;
         0 0 1 0;
         0 0 0 1];

% Rotation Transformation about x axis by alpha
T_R_x = [1          0           0 0;
         0 cos(alpha) -sin(alpha) 0;
         0 sin(alpha)  cos(alpha) 0;
         0          0           0 1];

% For a transformation FROM frame {i} TO frame {i-1}: A
T = T_R_z*T_T_z*T_T_x*T_R_x;

end

== matlab function QArm_Workspace_MB_2/To//From Simulation/Collision (Archive)/forward kinematics1 ==
  data: phi input; p4 output; R04 output
function [p4, R04] = qarmForwardKinematics(phi)

%% QUANSER_ARM_FPK
% v 4.0 - 4th June 2020

% REFERENCE: 
% Chapter 3. Forward Kinematics
% Robot Dynamics and Control 
% Spong, Vidyasagar
% 1989

% INPUTS:
% phi     : Alternate joint angles vector 4 x 1

% OUTPUTS:
% p4      : End-effector frame {4} position vector expressed in base frame {0}
% R04     : rotation matrix from end-effector frame {4} to base frame {0}

%% Manipulator parameters:
L1 = 0.1400;
L2 = 0.3500;
L3 = 0.0500;
L4 = 0.2500;
L5 = 0.1500;

%% Alternate parameters
l1 = L1;
l2 = sqrt(L2^2 + L3^2);
l3 = L4 + L5;
beta = atan(L3/L2);

%% From phi space to theta space 
theta = phi;
theta(1) = phi(1);
theta(2) = phi(2) + beta - pi/2;
theta(3) = phi(3) - beta;
theta(4) = phi(4);

%% Transformation matrices for all frames:

% T{i-1}{i} = quanser_arm_DH(  a, alpha,  d,     theta );
        T01 = quanser_arm_DH(  0, -pi/2, l1,  theta(1) );
        T12 = quanser_arm_DH( l2,     0,  0,  theta(2) );
        T23 = quanser_arm_DH(  0, -pi/2,  0,  theta(3) );
        T34 = quanser_arm_DH(  0,     0, l3,  theta(4) );

        T02 = T01*T12;
        T03 = T02*T23;
        T04 = T03*T34;

%% Position of end-effector Transformation

% Extract the Position vector 
% p1   = T01(1:3,4);
% p2   = T02(1:3,4);
% p3   = T03(1:3,4);
p4   = T04(1:3,4);

% Extract the Rotation matrix
% R01 = T01(1:3,1:3);
% R02 = T02(1:3,1:3);
% R03 = T03(1:3,1:3);
R04 = T04(1:3,1:3);

end

function T = quanser_arm_DH(a,alpha,d,theta)

%% QUANSER_ARM_DH
% v 1.0 - 26th March 2019

% REFERENCE: 
% Chapter 3. Forward and Inverse Kinematics
% Robot Modeling and Control 
% Spong, Hutchinson, Vidyasagar
% 2006

% INPUTS:
% a       :   translation  : along : x_{i}   : from : z_{i-1} : to : z_{i}
% alpha   :      rotation  : about : x_{i}   : from : z_{i-1} : to : z_{i}
% d       :   translation  : along : z_{i-1} : from : x_{i-1} : to : x_{i}
% theta   :      rotation  : about : z_{i-1} : from : x_{i-1} : to : x_{i}
% NOTE: Standard DH Parameters

% OUTPUTS:
% T       : transformation                   : from :     {i} : to : {i-1}

%%
% Rotation Transformation about z axis by theta
T_R_z = [cos(theta) -sin(theta) 0 0;
         sin(theta)  cos(theta) 0 0;
                  0           0 1 0;
                  0           0 0 1];
     
% Translation Transformation along z axis by d
T_T_z = [1 0 0 0;
         0 1 0 0;
         0 0 1 d;
         0 0 0 1];

% Translation Transformation along x axis by a
T_T_x = [1 0 0 a;
         0 1 0 0;
         0 0 1 0;
         0 0 0 1];

% Rotation Transformation about x axis by alpha
T_R_x = [1          0           0 0;
         0 cos(alpha) -sin(alpha) 0;
         0 sin(alpha)  cos(alpha) 0;
         0          0           0 1];

% For a transformation FROM frame {i} TO frame {i-1}: A
T = T_R_z*T_T_z*T_T_x*T_R_x;

end

== matlab function QArm_Workspace_MB_2/To//From Simulation/Collision (Archive)/inverse kinematics ==
  data: p input; gamma input; phi_optimal output; phi_prev input
function phi_optimal  = qarmInverseKinematics(p, gamma, phi_prev)

%% QUANSER_ARM_IPK
% v 4.0 - 4th June 2020

% REFERENCE: 
% Chapter 4. Inverse Kinematics
% Robot Dynamics and Control 
% Spong, Vidyasagar
% 1989

% INPUTS:
% p        : end-effector position vector expressed in base frame {0}
% gamma    : wrist rotation angle gamma

% OUTPUTS:
% phi_optimal : Best solution depending on phi_prev
% phi         : All four Inverse Kinematics solutions as a 4x4 matrix. 
%               Each col is a solution.

%% Manipulator parameters:
L1 = 0.1400;
L2 = 0.3500;
L3 = 0.0500;
L4 = 0.2500;
L5 = 0.1500;
beta = atan(L3/L2);

%% Alternate parameters
lambda1 = L1;
lambda2 = sqrt(L2^2 + L3^2);
lambda3 = L4 + L5;

%% Initialization
theta   = zeros(4, 4);
phi = zeros(4, 4);

%% Joint angle 2 and 3: 
% Equations:
    % lambda2 cos(theta2) + (-lambda3) sin(theta2 + theta3) = sqrt(x^2 + y^2)
    %   A     cos( 2    ) +     C      sin(   2   +    3  ) =    D
    
    % lambda2 sin(theta2) - (-lambda3) cos(theta2 + theta3) = lambda1 - z
    %   A     sin( 2    ) -     C      cos(   2   +    3  ) =    H

% Solution:
    A = lambda2;
    C = -lambda3;
    H =  lambda1 - p(3);
    D1 = -sqrt(p(1)^2 + p(2)^2);
    D2 = sqrt(p(1)^2 + p(2)^2);
    F = (D1^2 + H^2 - A^2 - C^2)/(2*A);

    theta(3,1) = 2*atan2( C + sqrt(C^2 - F^2) , F );
	theta(3,2) = 2*atan2( C - sqrt(C^2 - F^2) , F );
    theta(3,3) = 2*atan2( C + sqrt(C^2 - F^2) , F );
	theta(3,4) = 2*atan2( C - sqrt(C^2 - F^2) , F );

    M = A + C*sin(theta(3,1));
    N = -C*cos(theta(3,1));
    cos_term = (D1*M + H*N)/(M^2 + N^2);
    sin_term = (H - N*cos_term)/(M);
    theta(2,1) = atan2(sin_term, cos_term);

    M = A + C*sin(theta(3,2));
    N = -C*cos(theta(3,2));
    cos_term = (D1*M + H*N)/(M^2 + N^2);
    sin_term = (H - N*cos_term)/(M);
    theta(2,2) = atan2(sin_term, cos_term);

    M = A + C*sin(theta(3,3));
    N = -C*cos(theta(3,3));
    cos_term = (D2*M + H*N)/(M^2 + N^2);
    sin_term = (H - N*cos_term)/(M);
    theta(2,3) = atan2(sin_term, cos_term);

    M = A + C*sin(theta(3,4));
    N = -C*cos(theta(3,4));
    cos_term = (D2*M + H*N)/(M^2 + N^2);
    sin_term = (H - N*cos_term)/(M);
    theta(2,4) = atan2(sin_term, cos_term);


%% Joint angle 1:
% Equation:
    % y / x = tan(theta1);

% Solution
    theta(1,1) = atan2( p(2)/( lambda2 * cos( theta(2,1) ) - lambda3 * sin( theta(2,1) + theta(3,1) ) ) , p(1)/(  lambda2 * cos( theta(2,1) ) - lambda3 * sin( theta(2,1) + theta(3,1) )  ) );
    theta(1,2) = atan2( p(2)/( lambda2 * cos( theta(2,2) ) - lambda3 * sin( theta(2,2) + theta(3,2) ) ) , p(1)/(  lambda2 * cos( theta(2,2) ) - lambda3 * sin( theta(2,2) + theta(3,2) )  ) );
    theta(1,3) = atan2( p(2)/( lambda2 * cos( theta(2,3) ) - lambda3 * sin( theta(2,3) + theta(3,3) ) ) , p(1)/(  lambda2 * cos( theta(2,3) ) - lambda3 * sin( theta(2,3) + theta(3,3) )  ) );
    theta(1,4) = atan2( p(2)/( lambda2 * cos( theta(2,4) ) - lambda3 * sin( theta(2,4) + theta(3,4) ) ) , p(1)/(  lambda2 * cos( theta(2,4) ) - lambda3 * sin( theta(2,4) + theta(3,4) )  ) );
    
%% Remap theta back to phi
% phi(1) = theta(1);
% phi(2) = theta(2) - beta + pi/2;
% phi(3) = theta(3) + beta;
% phi(4) = theta(4);

phi(1,:) = theta(1,:);
phi(2,:) = theta(2,:) - beta + pi/2;
phi(3,:) = theta(3,:) + beta;
phi(4,:) = gamma;

phi = mod(phi + pi, 2*pi) - pi;

phi_optimal = phi(:,1);
if norm(phi_optimal - phi_prev) > norm(phi(:,2) - phi_prev)
    phi_optimal = phi(:,2);
end
if norm(phi_optimal - phi_prev) > norm(phi(:,3) - phi_prev)
    phi_optimal = phi(:,3);
end
if norm(phi_optimal - phi_prev) > norm(phi(:,4) - phi_prev)
    phi_optimal = phi(:,4);
end

end

== matlab function QArm_Workspace_MB_2/Virtual QArm/Manipulator Joint Plant - Queens/Dynamics ==
  data: pointLoadMass input; phi input; phi_d input; phi_dd input; tau output; Friction output
function [tau,Friction]   = f_QArm_Dynamics(pointLoadMass, phi, phi_d, phi_dd)
% Code updated by Leonam Pecly - November 10, 2021
% Based on code provided by Quanser

%%
g = 9.80665;

%% Manipulator parameters:
L1 = 0.1400;
L2 = 0.3500;
L3 = 0.0500;
L4 = 0.2500;
L5 = 0.1500;
beta = atan(L3/L2);

%% Alternate parameters
l1 = L1;                        % lambda 1
l2 = sqrt(L2^2 + L3^2);         % lambda 2
l3 = L4 + L5;                   % lambda 3

theta = phi - [0; pi/2-beta; beta; 0];
theta_d = phi_d;
theta_dd = phi_dd;

%% Dynamic Parameters
m1 = 0.7906;
m2 = 0.4591;
m3 = 0.269;
m4 = 0.257;
mL = pointLoadMass;
I1A = 1.489e-3;
I1L = 1;
I2A = 1.922e-4;
I2L = 9.61e-3;
I3A = 2.679e-4;
I3L = 2.069e-3;
I4A = 5.528e-4;
I4L = 1.12e-3;
% lc1 = l1/3;
% lc2 = l2/2;
% lc3 = L4/2;
% lc4 = L5/2;

lc1 = 0.0399;
lc2 = 0.1071;
lc3 = 0.1561;
lc4 = 0.0998;

%% Dynamic Matrices
% Inertia Matrix
M11 = I1A + m2*(l2 - lc2)^2*cos(theta(2))^2 + I2A*sin(theta(2))^2 + I2L*cos(theta(2))^2 + m3*l2^2*cos(theta(2))^2 + m3*lc3^2*sin(theta(2)+theta(3))^2 - 2*m3*l2*lc3*cos(theta(2))*sin(theta(2)+theta(3))...
    + I3L*sin(theta(2)+theta(3))^2 + I3A*cos(theta(2)+theta(3))^2 + m4*(l3 - lc4)^2*sin(theta(2)+theta(3))^2 + m4*l2^2*cos(theta(2))^2 - 2*m4*(l3-lc4)*l2*cos(theta(2))*sin(theta(2)+theta(3))...
    + I4L*sin(theta(2)+theta(3))^2 + I4A*cos(theta(2)+theta(3))^2 + mL*l3^2*sin(theta(2)+theta(3))^2 + mL*l2^2*cos(theta(2))^2 - 2*mL*l2*l3*cos(theta(2))*sin(theta(2)+theta(3));
M14 = -I4A*cos(theta(2)+theta(3));
M22 = m2*(l2-lc2)^2 + I2L + m3*l2^2+m3*lc3^2 - 2*m3*l2*lc3*sin(theta(3)) + I3L + m4*(l2+l3-lc4)^2 + I4L + mL*l2^2 + mL*l3^2 - 2*mL*l2*l3*sin(theta(3));
M23 = m3*lc3^2 - m3*lc3*l2*sin(theta(3)) + I3L + m4*(l3 - lc4 - l2*sin(theta(3)))*(l3 - lc4) + I4L - mL*(l3^2 - l2*l3*sin(theta(3)));
M32 = m3*lc3^2 - m3*lc3*l2*sin(theta(3)) + I3L + m4*(l3 - lc4 - l2*sin(theta(3)))*(l3 - lc4) + I4L - mL*(l3^2 - l2*l3*sin(theta(3)));
M33 = m3*lc3^2 + I3L + m4*(lc4 - l3)^2 + I4L + mL*l3^2;
M41 = -I4A*cos(theta(2)+theta(3));
M44 = I4A;
M = [M11, 0, 0, M14; 0, M22, M23, 0; 0, M32, M33, 0; M41, 0, 0, M44];

% Coriolis Matrix
B11 = -2*m2*(l2-lc2)^2*sin(theta(2))*cos(theta(2)) + 2*I2A*sin(theta(2))*cos(theta(2)) - 2*I2L*sin(theta(2))*cos(theta(2)) - 2*m3*l2^2*sin(theta(2))*cos(theta(2))...
     + 2*m3*lc3^2*sin(theta(2)+theta(3))*cos(theta(2)+theta(3)) + 2*m3*l2*lc3*sin(theta(2))*sin(theta(2)+theta(3)) - 2*m3*l2*lc3*cos(theta(2))*cos(theta(2)+theta(3))...
     + 2*I3L*sin(theta(2)+theta(3))*cos(theta(2)+theta(3)) - 2*I3A*sin(theta(2)+theta(3))*cos(theta(2)+theta(3)) + 2*m4*(l3 - lc4)^2*sin(theta(2)+theta(3))*cos(theta(2)+theta(3))...
     - 2*m4*l2^2*sin(theta(2))*cos(theta(2)) + 2*m4*(l3 - lc4)*l2*sin(theta(2))*sin(theta(2)+theta(3)) - 2*m4*(l3 - lc4)*l2*cos(theta(2))*cos(theta(2)+theta(3))...
     + 2*I4L*sin(theta(2)+theta(3))*cos(theta(2)+theta(3)) - 2*I4A*sin(theta(2)+theta(3))*cos(theta(2)+theta(3)) + 2*mL*l3^2*sin(theta(2)+theta(3))*cos(theta(2)+theta(3))...
     - 2*mL*l2^2*sin(theta(2))*cos(theta(2)) + 2*mL*l2*l3*sin(theta(2))*sin(theta(2)+theta(3)) - 2*mL*l2*l3*cos(theta(2))*cos(theta(2)+theta(3));
B12 =  2*m3*lc3^2*sin(theta(2)+theta(3))*cos(theta(2)+theta(3)) - 2*m3*l2*lc3*cos(theta(2))*cos(theta(2)+theta(3)) + 2*I3L*sin(theta(2)+theta(3))*cos(theta(2)+theta(3))...
     - 2*I3A*sin(theta(2)+theta(3))*cos(theta(2)+theta(3)) + 2*m4*(l3-lc4)^2*sin(theta(2)+theta(3))*cos(theta(2)+theta(3)) - 2*m4*(l3-lc4)*l2*cos(theta(2))*cos(theta(2)+theta(3))...
     + 2*I4L*sin(theta(2)+theta(3))*cos(theta(2)+theta(3)) - 2*I4A*sin(theta(2)+theta(3))*cos(theta(2)+theta(3)) + 2*mL*l3^2*sin(theta(2)+theta(3))*cos(theta(2)+theta(3))...
     - 2*mL*l2*l3*cos(theta(2))*cos(theta(2)+theta(3));
B15 =  I4A*sin(theta(2)+theta(3));
B16 =  I4A*sin(theta(2)+theta(3));
B23 = -I4A*sin(theta(2)+theta(3));
B24 = -2*m3*l2*lc3*cos(theta(3)) - 2*mL*l2*l3*cos(theta(3));
B33 = -I4A*sin(theta(2)+theta(3));
B41 =  I4A*sin(theta(2)+theta(3));
B42 =  I4A*sin(theta(2)+theta(3));
B = [B11, B12, 0, 0, B15, B16; 0, 0, B23, B24, 0, 0; 0, 0, B33, 0, 0, 0; B41, B42, 0, 0, 0, 0];

% Centrifugal Matrix
C21 = -(-m2*(l2-lc2)^2*sin(theta(2))*cos(theta(2)) + I2A*sin(theta(2))*cos(theta(2)) - I2L*sin(theta(2))*cos(theta(2)) - m3*l2^2*sin(theta(2))*cos(theta(2))...
     + m3*lc3^2*sin(theta(2)+theta(3))*cos(theta(2)+theta(3)) + m3*l2*lc3*sin(theta(2))*sin(theta(2)+theta(3)) - m3*l2*lc3*cos(theta(2))*cos(theta(2)+theta(3))  ...
     + I3L*sin(theta(2)+theta(3))*cos(theta(2)+theta(3)) - I3A*sin(theta(2)+theta(3))*cos(theta(2)+theta(3)) + m4*(l3-lc4)^2*sin(theta(2)+theta(3))*cos(theta(2)+theta(3))...
     - m4*l2^2*sin(theta(2))*cos(theta(2)) + m4*(l3-lc4)*l2*sin(theta(2))*sin(theta(2)+theta(3)) - m4*(l3-lc4)*l2*cos(theta(2))*cos(theta(2)+theta(3)) ...
     + I4L*sin(theta(2)+theta(3))*cos(theta(2)+theta(3)) - I4A*sin(theta(2)+theta(3))*cos(theta(2)+theta(3)) + mL*l3^2*sin(theta(2)+theta(3))*cos(theta(2)+theta(3))...
     - mL*l2^2*sin(theta(2))*cos(theta(2)) + mL*l2*l3*sin(theta(2))*sin(theta(2)+theta(3)) - mL*l2*l3*cos(theta(2))*cos(theta(2)+theta(3)));
C31 = -(m3*lc3^2*sin(theta(2)+theta(3))*cos(theta(2)+theta(3)) - m3*l2*lc3*cos(theta(2))*cos(theta(2)+theta(3)) + I3L*sin(theta(2)+theta(3))*cos(theta(2)+theta(3))...
      - I3A*sin(theta(2)+theta(3))*cos(theta(2)+theta(3)) + m4*(l3-lc4)^2*sin(theta(2)+theta(3))*cos(theta(2)+theta(3)) ...
      - m4*(l3-lc4)*l2*cos(theta(2))*cos(theta(2)+theta(3)) + I4L*sin(theta(2)+theta(3))*cos(theta(2)+theta(3)) - I4A*sin(theta(2)+theta(3))*cos(theta(2)+theta(3))... 
      + mL*l3^2*sin(theta(2)+theta(3))*cos(theta(2)+theta(3)) - mL*l2*l3*cos(theta(2))*cos(theta(2)+theta(3)));
C32 = m3*l2*lc3*cos(theta(3)) + mL*l2*l3*cos(theta(3));
C = [0, 0, 0, 0; C21, 0, 0, 0; C31, C32, 0, 0; 0, 0, 0, 0];

% Gravity Matrix

G2 = -g*(m2*(l2 - lc2)*cos(theta(2)) + m3*(l2*cos(theta(2)) - lc3*sin(theta(2)+theta(3))) + m4*(l2*cos(theta(2)) - (l3 - lc4)*sin(theta(2)+theta(3))) + mL*(l2*cos(theta(2)) - l3*sin(theta(2)+theta(3))) );
G3 = g*(m3*lc3*sin(theta(2)+theta(3)) + m4*(l3 - lc4)*sin(theta(2)+theta(3)) + mL*l3*sin(theta(2)+theta(3)) );

G = [0; G2; G3; 0];

%% Friction
% Friction = [0; 0; 0; 0];

Bv = [0.2119; 0.0457; 0.001; 0.008]; % Viscous coeffcients
Bc = [0.0838; 0.6701; 0.6156; 0.0275]; % Coulomb coeffcients

Friction = [Bv(1)*theta_d(1) + Bc(1)*sign(theta_d(1));...
             Bv(2)*theta_d(2) + Bc(2)*sign(theta_d(2));...
             Bv(3)*theta_d(3) + Bc(3)*sign(theta_d(3));...
             Bv(4)*theta_d(4) + Bc(4)*sign(theta_d(4))];  

%% Torque Computation (without Gravity)

B_signals = [theta_d(1) .* theta_d(2);...
             theta_d(1) .* theta_d(3);...
             theta_d(1) .* theta_d(4);...
             theta_d(2) .* theta_d(3);...
             theta_d(2) .* theta_d(4);...
             theta_d(3) .* theta_d(4);...
             ];

tau = M * theta_dd + B * B_signals + C * theta_d.^2 + G + Friction;
end

%%

== matlab function QArm_Workspace_MB_2/Virtual QArm/Manipulator Joint Plant - Queens/Gravitational Torque ==
  data: phi input; G output; payload input
function G  = fcn(phi, payload)

%% Manipulator Parameters and Initialization

% Manipulator natural link lengths
L1 = 0.1400;
L2 = 0.3500;
L3 = 0.0500;
L4 = 0.2500;
L5 = 0.1500;

% Manipulator bend angle at joint 3
beta = atan(L3/L2);

% Manipulator mathematical link lenghts
l1 = L1;
l2 = sqrt(L2^2 + L3^2);
l3 = L4 + L5;

% Phi-space to Theta-space
theta = phi;
theta(1) = phi(1);
theta(2) = phi(2) + beta - pi/2;
theta(3) = phi(3) - beta;
theta(4) = phi(4);

%% Dynamic Parameters (Inertias and Masses)

% Masses
mT = 1.75;
m1 = 0.3*mT*l1 / (l1 + l2 + l3);
m2 = mT*l2 / (l1 + l2 + l3);
m3 = mT*L4 / (l1 + l2 + l3);
m4 = mT*L5 / (l1 + l2 + l3);
mL = payload;

% Center of mass locations
% Note: lc1 is unused as the first link does not move linearly (v_1 = 0)
lc2 = l2/2;
lc3 = L4/2;
lc4 = L5/2;

%% Gravity Matrix

g = 9.81;
G2 = -g*(m2*(l2 - lc2)*cos(theta(2)) + m3*(l2*cos(theta(2)) - lc3*sin(theta(2)+theta(3))) + m4*(l2*cos(theta(2)) - (l3 - lc4)*sin(theta(2)+theta(3))) + mL*(l2*cos(theta(2)) - l3*sin(theta(2)+theta(3))) );
G3 = g*(m3*lc3*sin(theta(2)+theta(3)) + m4*(l3 - lc4)*sin(theta(2)+theta(3)) + mL*l3*sin(theta(2)+theta(3)) );

G = [0; G2; G3; 0];

== matlab function QArm_Workspace_MB_2/Virtual QArm/Manipulator Joint Plant - Queens/Subsystem/forward differential kinematics ==
  data: phi input size=[4]; J output size=[4,4]
function J  = qarmDifferentialKinematics(phi)

%% QUANSER_ARM_FPK
% v 4.0 - 4th June 2020

% REFERENCE: 
% Chapter 3. Forward Kinematics
% Robot Dynamics and Control 
% Spong, Vidyasagar
% 1989

% INPUTS:
% phi     : Alternate joint angles vector 4 x 1

% OUTPUTS:
% p4      : End-effector frame {4} position vector expressed in base frame {0}
% R04     : rotation matrix from end-effector frame {4} to base frame {0}

%% Manipulator parameters:
L1 = 0.1400;
L2 = 0.3500;
L3 = 0.0500;
L4 = 0.2500;
L5 = 0.1500;

%% Alternate parameters
l1 = L1;
l2 = sqrt(L2^2 + L3^2);
l3 = L4 + L5;
beta = atan(L3/L2);

%% From phi space to theta space 
theta = phi;
theta(1) = phi(1);
theta(2) = phi(2) + beta - pi/2;
theta(3) = phi(3) - beta;
theta(4) = phi(4);

%% Transformation matrices for all frames:

J = eye(4);
J(1,1) = - l2*sin(theta(1))*cos(theta(2)) + l3*sin(theta(1))*sin(theta(2)+theta(3)); 
J(1,2) = - l2*cos(theta(1))*sin(theta(2)) - l3*cos(theta(1))*cos(theta(2)+theta(3)); 
J(1,3) = - l3*cos(theta(1))*cos(theta(2)+theta(3)); 
J(1,4) = 0;
J(2,1) =   l2*cos(theta(1))*cos(theta(2)) - l3*cos(theta(1))*sin(theta(2)+theta(3)); 
J(2,2) = - l2*sin(theta(1))*sin(theta(2)) - l3*sin(theta(1))*cos(theta(2)+theta(3)); 
J(2,3) = - l3*sin(theta(1))*cos(theta(2)+theta(3));
J(2,4) = 0;
J(3,1) = 0; 
J(3,2) = - l2*cos(theta(2)) + l3*sin(theta(2)+theta(3)); 
J(3,3) =   l3*sin(theta(2)+theta(3));
J(3,4) = 0;
J(4,1) = 0;
J(4,2) = 0;
J(4,3) = 0;
J(4,4) = 1;

end
